simulink model "Example_2_Reduced_Order_Observer_Mdl"  (Simulink 7.1)
settings: Solver=ode23s  StartTime=0.0  StopTime=5  RelTol=1e-3
values from neighbouring files (symbols this model uses):
  A = sys.a    [Example_2_Control.m]    (also in Example_2_Discretization.m; Example_2_Disturbance_Estimation.m; Example_2_Integral_Control.m; Example_2_Prediction_Observer.m)
  A_11 = A(1,1)    [Example_2_Reduced_Order_Observer.m]
  A_12 = A(1,2:4)    [Example_2_Reduced_Order_Observer.m]
  A_21 = A(2:4,1)    [Example_2_Reduced_Order_Observer.m]
  A_22 = A(2:4,2:4)    [Example_2_Reduced_Order_Observer.m]
  a_ramp = 0.05    [Example_2_Control.m]    (also in Example_2_Discretization.m; Example_2_Integral_Control.m; Example_2_Prediction_Observer.m; Example_2_Reduced_Order_Observer.m)
  a_sin = 0.1    [Example_2_Control.m]    (also in Example_2_Discretization.m; Example_2_Integral_Control.m; Example_2_Prediction_Observer.m; Example_2_Reduced_Order_Observer.m)
  B = sys.b    [Example_2_Control.m]    (also in Example_2_Discretization.m; Example_2_Disturbance_Estimation.m; Example_2_Integral_Control.m; Example_2_Prediction_Observer.m)
  B_1 = B(1,1)    [Example_2_Reduced_Order_Observer.m]
  B_2 = B(2:4,1)    [Example_2_Reduced_Order_Observer.m]
  B_w = sys_d.b    [Example_2_Control.m]    (also in Example_2_Discretization.m; Example_2_Disturbance_Estimation.m; Example_2_Integral_Control.m; Example_2_Prediction_Observer.m)
  C = sys.c    [Example_2_Control.m]    (also in Example_2_Discretization.m; Example_2_Disturbance_Estimation.m; Example_2_Integral_Control.m; Example_2_Prediction_Observer.m)
  h = T_r/N_r    [Example_2_Control.m]    (also in Example_2_Discretization.m; Example_2_Disturbance_Estimation.m; Example_2_Integral_Control.m; Example_2_Prediction_Observer.m)
  L_r = L_r'    [Example_2_Reduced_Order_Observer.m]
  l_ramp = 0.05    [Example_2_Control.m]    (also in Example_2_Discretization.m; Example_2_Integral_Control.m; Example_2_Prediction_Observer.m; Example_2_Reduced_Order_Observer.m)
  l_sin = 5    [Example_2_Control.m]    (also in Example_2_Discretization.m; Example_2_Integral_Control.m; Example_2_Prediction_Observer.m; Example_2_Reduced_Order_Observer.m)
  v = 40/3.6    (= 11.1111111111)    [Example_2_Control.m]    (also in Example_2_Discretization.m; Example_2_Disturbance_Estimation.m; Example_2_Integral_Control.m; Example_2_Prediction_Observer.m)
  x_0 = [0; 0; 0; 0]    [Example_2_Analysis.m]    (also in Example_2_Control.m = [25*9.81/k_s; 0; 25*9.81/k_u; 0]; Example_2_Discretization.m = [25*9.81/k_s; 0; 25*9.81/k_u; 0]; Example_2_Disturbance_Estimation.m; Example_2_Integral_Control.m)
  x_0_red = [0; 0; 0]    [Example_2_Reduced_Order_Observer.m]
libraries: simulink x1
settings Model: Creator=d_goerges  LastModifiedBy=d_goerges
settings DataIOCC: Refine=10
settings OptimizationCC: InitFltsAndDblsToZero=off
settings DebuggingCC: FcnCallInpInsideContextMsg=Enable All  StrictBusMsg=ErrorLevel1
settings GRTTargetCC: CPPClassGenCompliant=off

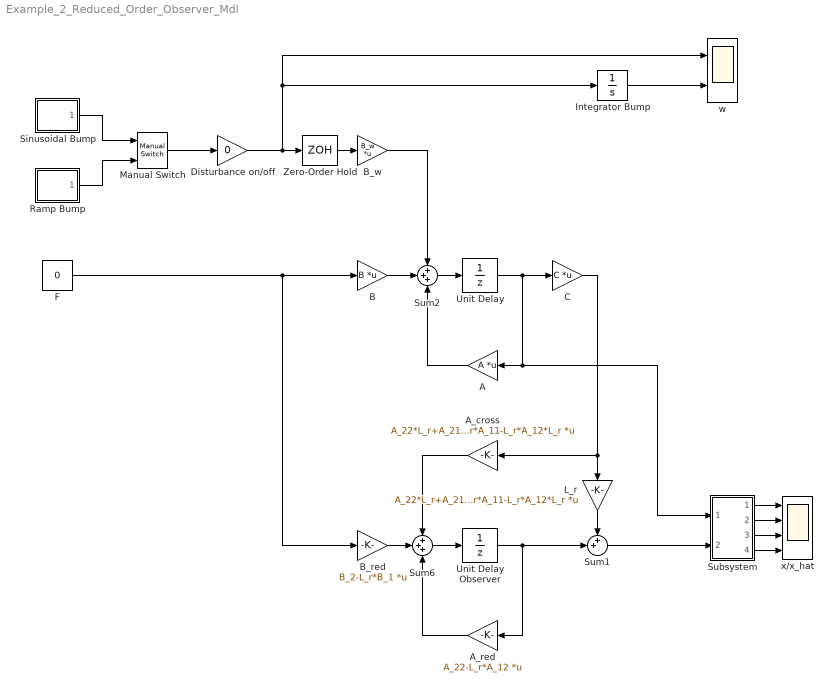
== system Example_2_Reduced_Order_Observer_Mdl ==
  A : Gain  Orientation=left  Gain=A  Multiplication=Matrix(K*u)
  A_cross : Gain  Orientation=left  Gain=A_22*L_r+A_21-L_r*A_11-L_r*A_12*L_r  Multiplication=Matrix(K*u)
  A_red : Gain  Orientation=left  Gain=A_22-L_r*A_12  Multiplication=Matrix(K*u)
  B : Gain  Gain=B  Multiplication=Matrix(K*u)
  B_red : Gain  Gain=B_2-L_r*B_1  Multiplication=Matrix(K*u)
  B_w : Gain  Gain=B_w  Multiplication=Matrix(K*u)  SampleTime=h
  C : Gain  Gain=C  Multiplication=Matrix(K*u)
  Disturbance on/off : Gain  Gain=0
  F : Constant  Value=0
  Integrator Bump : Integrator
  L_r : Gain  Orientation=down  Gain=A_22*L_r+A_21-L_r*A_11-L_r*A_12*L_r  Multiplication=Matrix(K*u)
  Manual Switch : simulink/Signal Routing/Manual Switch  sw=1  action=0  varsize=off
  Ramp Bump : Subsystem
  Sinusoidal Bump : Subsystem
  Subsystem : Subsystem
  Sum1 : Sum  Inputs=++|
  Sum2 : Sum  Inputs=+++
  Sum6 : Sum  Inputs=+++
  Unit Delay : UnitDelay  X0=x_0  SampleTime=h
  Unit Delay Observer : UnitDelay  X0=x_0_red  SampleTime=h
  Zero-Order Hold : ZeroOrderHold  SampleTime=h
  w : Scope  NumInputPorts=2
      settings: YMin=-5~-5  YMax=5~5  SaveName=ScopeData2
  x/x_hat : Scope  NumInputPorts=4
      settings: TimeRange=5  YMin=-0.03~-0.4~-0.004~-0.2  YMax=0.05~0.3~0.01~0.5  SaveName=ScopeData3
  wires:
  Sum2/1 -> Unit Delay/1
  B/1 -> Sum2/2
  A/1 -> Sum2/3
  B_w/1 -> Sum2/1
  Subsystem/1(Out1) -> x/x_hat/1
  Subsystem/2(Out2) -> x/x_hat/2
  Subsystem/3(Out3) -> x/x_hat/3
  Subsystem/4(Out4) -> x/x_hat/4
  Manual Switch/1 -> Disturbance on/off/1
  Unit Delay/1 -> C/1, A/1, Subsystem/1(In1)
  Sinusoidal Bump/1(z_r_dot) -> Manual Switch/1
  Ramp Bump/1(z_r_dot) -> Manual Switch/2
  Integrator Bump/1 -> w/2
  Sum6/1 -> Unit Delay Observer/1
  Unit Delay Observer/1 -> A_red/1, Sum1/2
  F/1 -> B_red/1, B/1
  B_red/1 -> Sum6/2
  A_red/1 -> Sum6/3
  A_cross/1 -> Sum6/1
  Zero-Order Hold/1 -> B_w/1
  C/1 -> A_cross/1, L_r/1
  L_r/1 -> Sum1/1
  Sum1/1 -> Subsystem/2(In2)
  Disturbance on/off/1 -> w/1, Integrator Bump/1, Zero-Order Hold/1

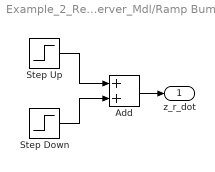
== system Example_2_Reduced_Order_Observer_Mdl/Ramp Bump ==
  Add : Sum
  Step Down : Step  Time=l_ramp/v  After=-a_ramp/l_ramp*v  SampleTime=0
  Step Up : Step  Time=0  After=a_ramp/l_ramp*v  SampleTime=0
  z_r_dot : Outport
  wires:
  Step Up/1 -> Add/1
  Step Down/1 -> Add/2
  Add/1 -> z_r_dot/1

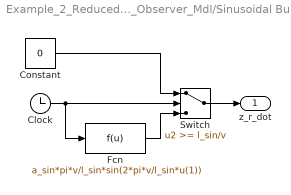
== system Example_2_Reduced_Order_Observer_Mdl/Sinusoidal Bump ==
  Clock : Clock
  Constant : Constant  Value=0
  Fcn : Fcn  Expr=a_sin*pi*v/l_sin*sin(2*pi*v/l_sin*u(1))
  Switch : Switch  Threshold=l_sin/v
  z_r_dot : Outport
  wires:
  Switch/1 -> z_r_dot/1
  Fcn/1 -> Switch/3
  Constant/1 -> Switch/1
  Clock/1 -> Fcn/1, Switch/2

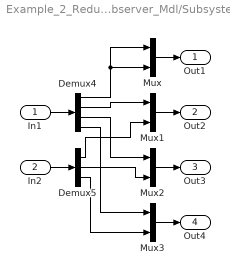
== system Example_2_Reduced_Order_Observer_Mdl/Subsystem ==
  In1 : Inport
  In2 : Inport  Port=2
  Demux4 : Demux
  Demux5 : Demux  Outputs=3
  Mux{,1..3} (4 alike) : Mux  Inputs=2
  Out1 : Outport
  Out2 : Outport  Port=2
  Out3 : Outport  Port=3
  Out4 : Outport  Port=4
  wires:
  Demux4/1 -> Mux/1, Mux/2
  Demux4/2 -> Mux1/1
  Demux4/3 -> Mux2/1
  Demux4/4 -> Mux3/1
  Mux/1 -> Out1/1
  In1/1 -> Demux4/1
  Mux1/1 -> Out2/1
  In2/1 -> Demux5/1
  Mux2/1 -> Out3/1
  Mux3/1 -> Out4/1
  Demux5/1 -> Mux1/2
  Demux5/2 -> Mux2/2
  Demux5/3 -> Mux3/2
